simulink model "demo"  (R2016a)
settings: Solver=ode45  StartTime=0.0  StopTime=100  RelTol=1e-3
values from neighbouring files (symbols this model uses):
  P = computeGainsAerosonde(T_phi_delta_a,T_v_delta_r,T_theta_delta_e,T_Va_theta,T_Va_delta_t,P)    [run_autopilot.m]
  U_trim = [-0.0594; 0.0005; -0.0010; 0.0978]    [run_autopilot.m]
  x0 = X_trim    [run_autopilot.m]
  X_trim = [0; 0; -100.0000; 0.9993; -0.0011; 0.0332; 0.0186; 35.7388;             -0.0122; 2.3784; 0; 0; 0; -0.0300; 0; -0.0294; 0; 0.0978]    [run_autopilot.m]
undefined symbols (not defined in the file or in its folder): Earth, h_ref, lat0, lon0, T_elevon2ailelev, WGS84
undefined symbols (not defined in the file): param
libraries: simulink_extras x7, simulink x5, aerolibfltsims x4, X8_lib x3, aerolibactuator x3, aerolibanimutils x2, aerolibtransform2 x1, aerolibutil x1
settings Model: Creator=krisgry  LastModifiedBy=andreanv
settings DataIOCC: LimitDataPoints=on  SaveFormat=Array
settings DebuggingCC: AllowSymbolicDim=off
settings HardwareCC: ProdBitPerPointer=32  ProdLargestAtomicFloat=None  ProdIntDivRoundTo=Undefined  ProdEndianess=Unspecified  ProdWordSize=32  ProdHWDeviceType=32-bit Generic
settings ModelReferenceCC: PropagateSignalLabelsOutOfModel=off
settings ConfigComp: CovModelRefEnable=Off

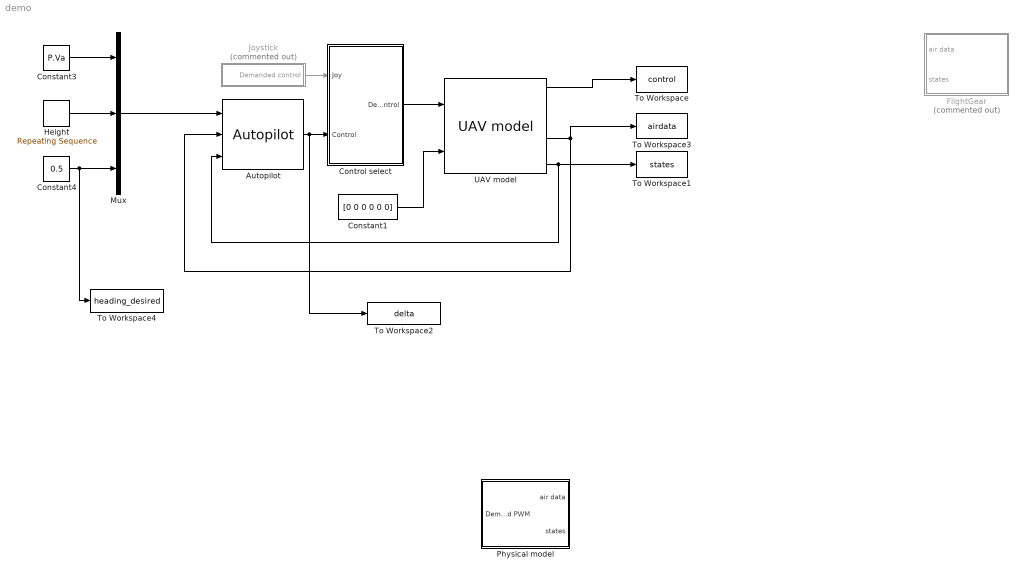
== system demo ==
  Autopilot : X8_lib/Autopilot  param=param  X_trim=X_trim  U_trim=U_trim
  Constant1 : Constant  Value=[0 0 0 0 0 0]
  Constant3 : Constant  Value=P.Va
  Constant4 : Constant  Value=0.5
  Control select : Subsystem
  FlightGear : Subsystem  Commented=on
  Height : simulink/Sources/Repeating Sequence  rep_seq_t=[0 1]  rep_seq_y=[-100 -100]
  Joystick : Subsystem  Commented=on
  Mux : Mux  Inputs=3
  Physical model : Subsystem
  To Workspace : ToWorkspace  VariableName=control  SaveFormat=Timeseries  SampleTime=-1
  To Workspace1 : ToWorkspace  VariableName=states  SaveFormat=Timeseries  SampleTime=-1
  To Workspace2 : ToWorkspace  VariableName=delta  SaveFormat=Timeseries  SampleTime=-1
  To Workspace3 : ToWorkspace  VariableName=airdata  SaveFormat=Timeseries  SampleTime=-1
  To Workspace4 : ToWorkspace  VariableName=heading_desired  SaveFormat=Timeseries  SampleTime=-1
  UAV model : X8_lib/UAV model  param=param  pos0=X_trim(1:3)'  quat0=X_trim(4:7)'  vel0=X_trim(8:10)'  rate0=X_trim(11:13)'  servoR_pos0=X_trim(14)  servoR_vel0=X_trim(15)  servoL_pos0=X_trim(16)  servoL_vel0=X_trim(17)  motor_speed0=X_trim(18)
  wires:
  Joystick/1(Demanded control) -> Control select/1(Joy)
  Autopilot/1 -> To Workspace2/1, Control select/2(Control)
  Mux/1 -> Autopilot/1
  Height/1 -> Mux/2
  Constant3/1 -> Mux/1
  Constant4/1 -> Mux/3, To Workspace4/1
  Control select/1(Demanded control) -> UAV model/1
  Constant1/1 -> UAV model/2
  UAV model/4 -> To Workspace1/1, Autopilot/3
  UAV model/3 -> To Workspace3/1, Autopilot/2
  UAV model/1 -> To Workspace/1

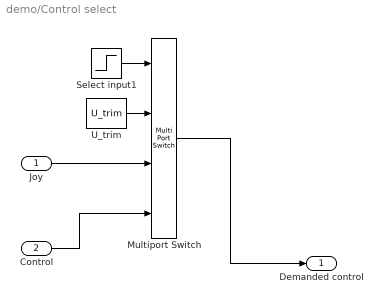
== system demo/Control select ==
  Joy : Inport
  Control : Inport  Port=2
  Multiport Switch : MultiPortSwitch
  Select input1 : Step  Time=0  Before=1  After=3  SampleTime=0
  U_trim : Constant  Value=U_trim
  Demanded control : Outport
  wires:
  Control/1 -> Multiport Switch/4
  Multiport Switch/1 -> Demanded control/1
  U_trim/1 -> Multiport Switch/2
  Joy/1 -> Multiport Switch/3
  Select input1/1 -> Multiport Switch/1

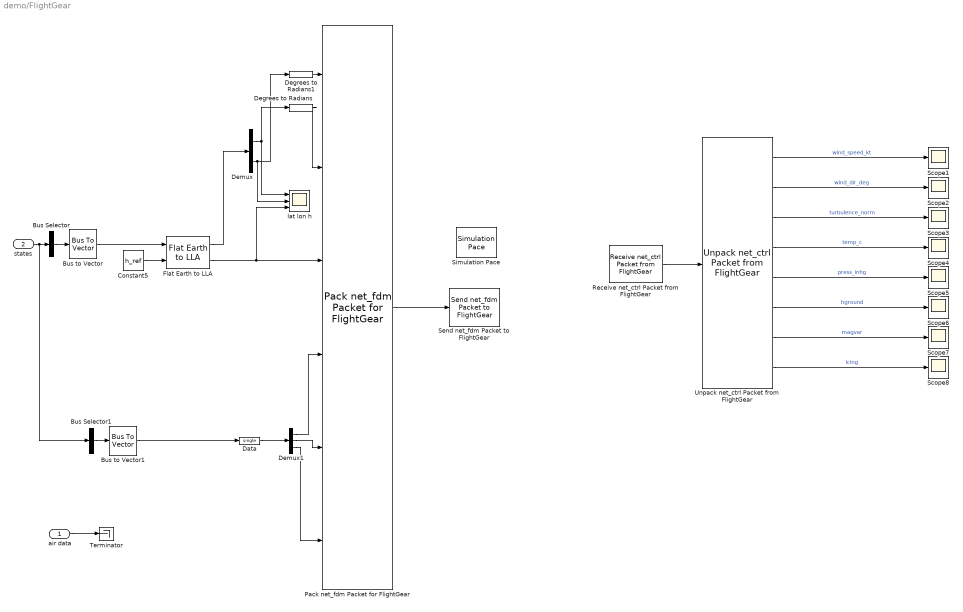
== system demo/FlightGear ==
  air data : Inport
  states : Inport  Port=2
  Bus Selector : BusSelector  OutputSignals=Position.p_N,Position.p_E,Position.p_D  OutputAsBus=on
  Bus Selector1 : BusSelector  OutputSignals=Attitude  OutputAsBus=on
  Bus to Vector : BusToVector
  Bus to Vector1 : BusToVector
  Constant5 : Constant  Value=h_ref
  Data : DataTypeConversion  OutDataTypeStr=single
  Degrees to Radians : simulink_extras/Transformations/Degrees to Radians
  Degrees to Radians1 : simulink_extras/Transformations/Degrees to Radians
  Demux : Demux  Outputs=2
  Demux1 : Demux  Outputs=3
  Flat Earth to LLA : aerolibtransform2/Flat Earth to LLA  units=Metric (MKS)  ptype=Earth (WGS84)  F=1/298.257223563  R=6378137  LL0=[lat0 lon0]  psi=0
  Pack net_fdm Packet for FlightGear : aerolibfltsims/Pack net_fdm Packet for FlightGear  FlightGearVersion=v2.12  ShowPositionAttitudeInputs=on  ShowVelocityAccelerationInputs=off  ShowControlSurfacePositionInputs=off  ShowEngineFuelInputs=off  ShowLandingGearInputs=off  ShowEnvironmentInputs=off  SampleTime=1/30
  Receive net_ctrl Packet from FlightGear : aerolibfltsims/Receive net_ctrl Packet from FlightGear  FlightGearVersion=v2.12  ReceiveAddress=129.241.154.119  ReceivePort=5505  ReceiveWidth=744  varLen=off  SampleTime=1/30  packetFlag=off
      settings: AttributesFormatString=Version Selected:\n%<FlightGearVersion>
  Scope{1..8} (8 alike) : Scope
  Send net_fdm Packet to FlightGear : aerolibfltsims/Send net_fdm Packet to FlightGear  DestinationIpAddress=129.241.154.119  DestinationPort=5502  LocalIpPort=-1  varLen=off  SampleTime=1/30
  Simulation Pace : aerolibanimutils/Simulation Pace  SimulationPace=1  SleepMode=MATLAB Thread  OutputPaceError=off  SampleTime=1/30
      settings: AttributesFormatString=%<SimulationPace> sec/sec
  Terminator : Terminator
  Unpack net_ctrl Packet from FlightGear : aerolibfltsims/Unpack net_ctrl Packet from FlightGear  FlightGearVersion=v2.12  ShowControlSurfacePositionOutputs=off  ShowEngineFuelOutputs=off  ShowLandingGearOutputs=off  ShowAvionicOutputs=off  ShowEnvironmentOutputs=on  SampleTime=1/30
      settings: AttributesFormatString=Version Selected: %<FlightGearVersion>
  lat lon h : Scope  NumInputPorts=3
  wires:
  Pack net_fdm Packet for FlightGear/1 -> Send net_fdm Packet to FlightGear/1
  Demux1/1 -> Pack net_fdm Packet for FlightGear/4
  Demux1/2 -> Pack net_fdm Packet for FlightGear/5
  Demux1/3 -> Pack net_fdm Packet for FlightGear/6
  Demux/2 -> lat lon h/2, Degrees to Radians1/1
  Demux/1 -> Degrees to Radians/1, lat lon h/1
  Data/1 -> Demux1/1
  Degrees to Radians/1 -> Pack net_fdm Packet for FlightGear/2
  Degrees to Radians1/1 -> Pack net_fdm Packet for FlightGear/1
  Unpack net_ctrl Packet from FlightGear/1 -> Scope1/1  "wind_speed_kt"
  Receive net_ctrl Packet from FlightGear/1 -> Unpack net_ctrl Packet from FlightGear/1
  Unpack net_ctrl Packet from FlightGear/2 -> Scope2/1  "wind_dir_deg"
  Unpack net_ctrl Packet from FlightGear/3 -> Scope3/1  "turbulence_norm"
  Unpack net_ctrl Packet from FlightGear/4 -> Scope4/1  "temp_c"
  Unpack net_ctrl Packet from FlightGear/5 -> Scope5/1  "press_inhg"
  Unpack net_ctrl Packet from FlightGear/6 -> Scope6/1  "hground"
  Unpack net_ctrl Packet from FlightGear/7 -> Scope7/1  "magvar"
  Unpack net_ctrl Packet from FlightGear/8 -> Scope8/1  "icing"
  air data/1 -> Terminator/1
  Constant5/1 -> Flat Earth to LLA/2
  Flat Earth to LLA/1 -> Demux/1
  Bus Selector/1 -> Bus to Vector/1
  Bus to Vector/1 -> Flat Earth to LLA/1
  Flat Earth to LLA/2 -> lat lon h/3, Pack net_fdm Packet for FlightGear/3
  Bus Selector1/1 -> Bus to Vector1/1
  Bus to Vector1/1 -> Data/1
  states/1 -> Bus Selector1/1, Bus Selector/1

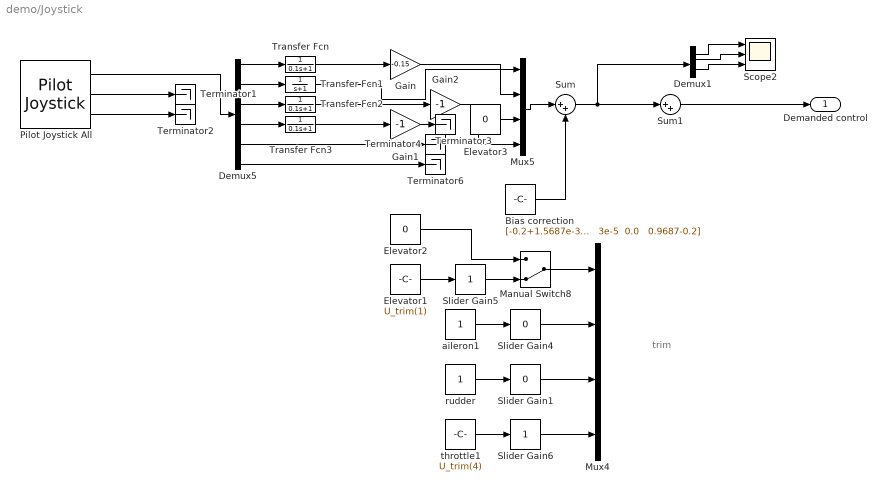
== system demo/Joystick ==
  note: trim
  Bias correction : Constant  Value="[-0.2+1.5687e-3   3e-5  0.0   0.9687-0.2]"
  Demux1 : Demux
  Demux5 : Demux  Outputs=6
  Elevator1 : Constant  Value=U_trim(1)
  Elevator2 : Constant  Value=0
  Elevator3 : Constant  Value=0
  Gain : Gain  Gain=-0.15
  Gain1 : Gain  Gain=-1
  Gain2 : Gain  Gain=-1
  Manual Switch8 : ManualSwitch  CurrentSetting=0
  Mux4 : Mux
  Mux5 : Mux
  Pilot Joystick All : aerolibanimutils/Pilot Joystick  JoystickID=Joystick1  OutputConfiguration=AllOutputs  SampleTime=1/30
  Scope2 : Scope  NumInputPorts=3
  Slider Gain1 : simulink/Math Operations/Slider Gain  low=-1  gain=0  high=1
  Slider Gain4 : simulink/Math Operations/Slider Gain  low=-1  gain=0  high=1
  Slider Gain5 : simulink/Math Operations/Slider Gain  low=-1  gain=1  high=1
  Slider Gain6 : simulink/Math Operations/Slider Gain  low=0  gain=1  high=2
  Sum : Sum  Inputs=|++
  Sum1 : Sum  Inputs=|++
  Terminator{1..4,6} (5 alike) : Terminator
  Transfer Fcn : TransferFcn  Denominator=[0.1 1]
  Transfer Fcn1 : TransferFcn  Denominator=[1 1]
  Transfer Fcn2 : TransferFcn  Denominator=[0.1 1]
  Transfer Fcn3 : TransferFcn  Denominator=[0.1 1]
  aileron1 : Constant
  rudder : Constant
  throttle1 : Constant  Value=U_trim(4)
  Demanded control : Outport
  wires:
  Gain/1 -> Mux5/2
  Demux5/5 -> Terminator4/1
  Demux5/1 -> Transfer Fcn/1
  Demux5/6 -> Terminator6/1
  Demux5/4 -> Transfer Fcn3/1
  Pilot Joystick All/3 -> Terminator2/1
  Pilot Joystick All/2 -> Terminator1/1
  Gain1/1 -> Terminator3/1
  Demux5/3 -> Transfer Fcn2/1
  Mux5/1 -> Sum/1
  Bias correction/1 -> Sum/2
  Gain2/1 -> Mux5/4
  Demux1/1 -> Scope2/1
  Demux1/2 -> Scope2/2
  Sum/1 -> Sum1/1, Demux1/1
  Elevator1/1 -> Slider Gain5/1
  aileron1/1 -> Slider Gain4/1
  Slider Gain4/1 -> Mux4/2
  Slider Gain6/1 -> Mux4/4
  Manual Switch8/1 -> Mux4/1
  Slider Gain5/1 -> Manual Switch8/2
  Elevator2/1 -> Manual Switch8/1
  Sum1/1 -> Demanded control/1
  throttle1/1 -> Slider Gain6/1
  Demux1/4 -> Scope2/3
  Elevator3/1 -> Mux5/3
  rudder/1 -> Slider Gain1/1
  Slider Gain1/1 -> Mux4/3
  Demux5/2 -> Transfer Fcn1/1
  Pilot Joystick All/1 -> Demux5/1
  Transfer Fcn/1 -> Gain/1
  Transfer Fcn1/1 -> Mux5/1
  Transfer Fcn2/1 -> Gain2/1
  Transfer Fcn3/1 -> Gain1/1

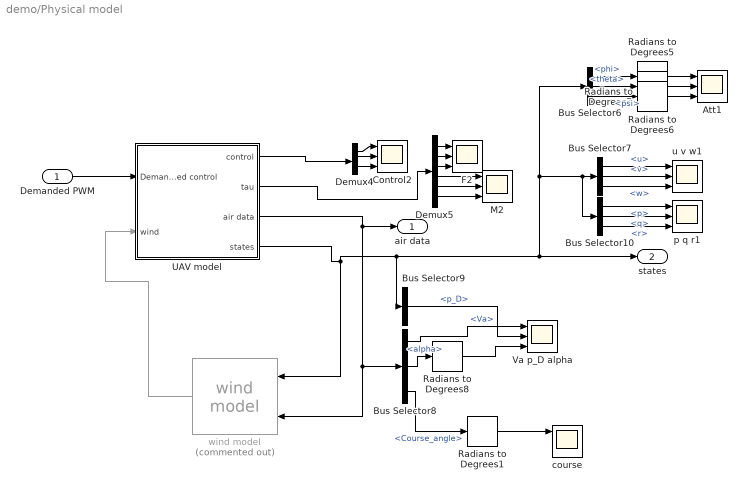
== system demo/Physical model ==
  Demanded PWM : Inport
  Att1 : Scope  NumInputPorts=3
  Bus Selector10 : BusSelector  OutputSignals=AngularVelocity.p,AngularVelocity.q,AngularVelocity.r
  Bus Selector6 : BusSelector  OutputSignals=Attitude.phi,Attitude.theta,Attitude.psi
  Bus Selector7 : BusSelector  OutputSignals=Velocity.u,Velocity.v,Velocity.w
  Bus Selector8 : BusSelector  OutputSignals=Va,alpha,Course_angle
  Bus Selector9 : BusSelector  OutputSignals=Position.p_D
  Control2 : Scope  NumInputPorts=3
  Demux4 : Demux
  Demux5 : Demux  Outputs=6
  F2 : Scope  NumInputPorts=3
  M2 : Scope  NumInputPorts=3
  Radians to Degrees{1,5..8} (5 alike) : simulink_extras/Transformations/Radians to Degrees
  UAV model : Subsystem  AncestorBlock=X8_lib/UAV model  mask{param=param, pos0=X_trim(1:3)', quat0=X_trim(4:7)', vel0=X_trim(8:10)', rate0=X_trim(11:13)', servoR_pos0=X_trim(14), servoR_vel0=X_trim(15), servoL_pos0=X_trim(16), servoL_vel0=X_trim(17), motor_speed0=X_trim(18)}
      mask prompts: param "UAV model"; pos0 "NED Position"; quat0 "Quaternion"; vel0 "Velocity"; rate0 "Angular Velocity"; servoR_pos0 "Right servo deflection"; servoR_vel0 "Right servo velocity"; servoL_pos0 "Left servo deflection"; servoL_vel0 "Left servo velocity"; motor_speed0 "Motor speed"
      mask help:
      | UAV model can be either 'x8_param' or 'aerosonde'
      |
      | # Inputs:
      | Demanded control: a 4x1 vector consisting of [elevator, aileron, rudder, throttle]
      | wind: a 6x1 vector consisting of the wind+gust in NED, and the body rate gusts: [N,E,D,p,q,r]
      |
      | # Outputs:
      | control: the control vector after it has been passed through the actuator model
      | tau: a 6x1 force/moment vector: [Fx,Fy,Fz,l,m,n]
      | airdata: a 10-element bus with airspeed, alpha, beta ... see bus_definitions.m
      | states: a bus consisting of 6 buses: position, attitude, quaternion, velocity, angular velocity, acceleration. See bus_definitions.m
      mask init:
      | %bus_defintions;
      | if(~exist('P') || ~isfield(P,'b'))
      |     init;
      | end
      mask DialogControl Container3 Prompt: Initial conditions
      mask Display:
      | image('X8.png')
      | port_label('output',1,'\delta','texmode','on')
      | port_label('output',2,'\tau','texmode','on')
      | port_label('output',3,'AirData','texmode','on')
      | port_label('output',4,'States','texmode','on')
      | port_label('input',1,'\delta_{demand}','texmode','on')
      | port_label('input',2,'Wind','texmode','on')
  Va p_D alpha : Scope  NumInputPorts=3
  course : Scope  NumInputPorts=3
  p q r1 : Scope  NumInputPorts=3
  u v w1 : Scope  NumInputPorts=3
  wind model : X8_lib/wind model  Commented=on  wind_speed=0  wind_dir=0  wind_start_time=0  param='x8_param'
  air data : Outport
  states : Outport  Port=2
  wires:
  Demux5/1 -> F2/1
  Demux5/2 -> F2/2
  Demux5/3 -> F2/3
  Demux5/4 -> M2/1
  Demux5/5 -> M2/2
  Demux5/6 -> M2/3
  Bus Selector7/1 -> u v w1/1  "<u>"
  Bus Selector7/2 -> u v w1/2  "<v>"
  Bus Selector7/3 -> u v w1/3  "<w>"
  Bus Selector6/1 -> Radians to Degrees5/1  "<phi>"
  Bus Selector6/3 -> Radians to Degrees7/1  "<psi>"
  Bus Selector6/2 -> Radians to Degrees6/1  "<theta>"
  Radians to Degrees5/1 -> Att1/1
  Radians to Degrees6/1 -> Att1/2
  Radians to Degrees7/1 -> Att1/3
  Bus Selector8/1 -> Va p_D alpha/1  "<Va>"
  Bus Selector9/1 -> Va p_D alpha/2  "<p_D>"
  Bus Selector8/2 -> Radians to Degrees8/1  "<alpha>"
  Radians to Degrees8/1 -> Va p_D alpha/3
  Demux4/4 -> Control2/3
  Demux4/2 -> Control2/2
  Demux4/1 -> Control2/1
  Bus Selector10/1 -> p q r1/1  "<p>"
  Bus Selector10/2 -> p q r1/2  "<q>"
  Bus Selector10/3 -> p q r1/3  "<r>"
  UAV model/3(air data) -> air data/1, wind model/2, Bus Selector8/1
  UAV model/4(states) -> wind model/1, Bus Selector9/1, Bus Selector6/1, Bus Selector7/1, Bus Selector10/1, states/1
  UAV model/2(tau) -> Demux5/1
  UAV model/1(control) -> Demux4/1
  wind model/1 -> UAV model/2(wind)
  Demanded PWM/1 -> UAV model/1(Demanded control)
  Bus Selector8/3 -> Radians to Degrees1/1  "<Course_angle>"
  Radians to Degrees1/1 -> course/1

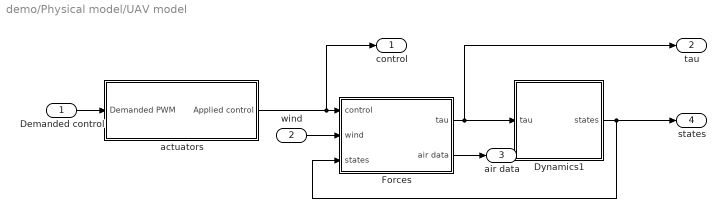
== system demo/Physical model/UAV model ==
  Demanded control : Inport
  wind : Inport  Port=2  PortDimensions=6
  Dynamics1 : Subsystem
  Forces : Subsystem
  actuators : Subsystem
  control : Outport
  tau : Outport  Port=2
  air data : Outport  Port=3  OutDataTypeStr=Bus: AirData
  states : Outport  Port=4  OutDataTypeStr=Bus: States
  wires:
  actuators/1(Applied control) -> Forces/1(control), control/1
  Forces/2(air data) -> air data/1
  Dynamics1/1(states) -> Forces/3(states), states/1
  Forces/1(tau) -> Dynamics1/1(tau), tau/1
  Demanded control/1 -> actuators/1(Demanded PWM)
  wind/1 -> Forces/2(wind)

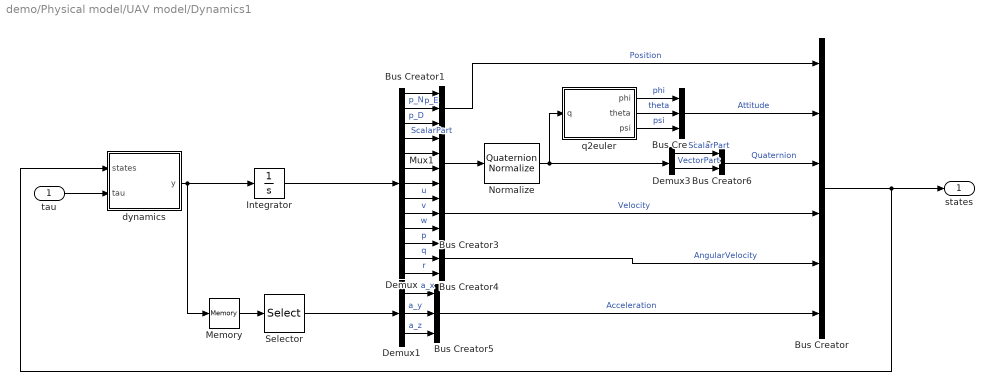
== system demo/Physical model/UAV model/Dynamics1 ==
  tau : Inport
  Bus Creator : BusCreator  Inputs=6  OutDataTypeStr=Bus: States
  Bus Creator1 : BusCreator  Inputs=3  OutDataTypeStr=Bus: Position
  Bus Creator2 : BusCreator  Inputs=3  OutDataTypeStr=Bus: Attitude
  Bus Creator3 : BusCreator  Inputs=3  OutDataTypeStr=Bus: Velocity
  Bus Creator4 : BusCreator  Inputs=3  OutDataTypeStr=Bus: AngularVelocity
  Bus Creator5 : BusCreator  Inputs=3  OutDataTypeStr=Bus: Acceleration
  Bus Creator6 : BusCreator  Inputs=2  OutDataTypeStr=Bus: Quaternion
  Demux : Demux  Outputs=13
  Demux1 : Demux  Outputs=3
  Demux3 : Demux  Outputs=[1,3]
  Integrator : Integrator  InitialCondition=[pos0,quat0,vel0,rate0]%x0(1:13)
  Memory : Memory
  Mux1 : Mux
  Normalize : aerolibutil/Quaternion Normalize
  Selector : Selector  InputPortWidth=13  IndexOptions=Index vector (dialog)  Indices=8:10  OutputSizes=1
  dynamics : MATLAB Function  TreatAsAtomicUnit=on
  q2euler : MATLAB Function  TreatAsAtomicUnit=on
  states : Outport
  wires:
  Memory/1 -> Selector/1
  Mux1/1 -> Normalize/1
  Bus Creator2/1 -> Bus Creator/2  "Attitude"
  Demux/4 -> Mux1/1  "ScalarPart"
  Bus Creator6/1 -> Bus Creator/3  "Quaternion"
  Demux3/2 -> Bus Creator6/2  "VectorPart"
  Demux3/1 -> Bus Creator6/1  "ScalarPart"
  Integrator/1 -> Demux/1
  Normalize/1 -> Demux3/1, q2euler/1(q)
  Demux/5 -> Mux1/2
  Demux/7 -> Mux1/4
  Demux/6 -> Mux1/3
  Demux1/3 -> Bus Creator5/3  "a_z"
  Demux1/2 -> Bus Creator5/2  "a_y"
  Demux1/1 -> Bus Creator5/1  "a_x"
  Selector/1 -> Demux1/1
  Bus Creator5/1 -> Bus Creator/6  "Acceleration"
  Bus Creator4/1 -> Bus Creator/5  "AngularVelocity"
  Bus Creator1/1 -> Bus Creator/1  "Position"
  Bus Creator3/1 -> Bus Creator/4  "Velocity"
  Demux/12 -> Bus Creator4/2  "q"
  Demux/13 -> Bus Creator4/3  "r"
  Demux/11 -> Bus Creator4/1  "p"
  Demux/9 -> Bus Creator3/2  "v"
  Demux/8 -> Bus Creator3/1  "u"
  Demux/10 -> Bus Creator3/3  "w"
  q2euler/1(phi) -> Bus Creator2/1  "phi"
  q2euler/3(psi) -> Bus Creator2/3  "psi"
  q2euler/2(theta) -> Bus Creator2/2  "theta"
  Demux/1 -> Bus Creator1/1  "p_N"
  Demux/3 -> Bus Creator1/3  "p_D"
  Demux/2 -> Bus Creator1/2  "p_E"
  Bus Creator/1 -> dynamics/1(states), states/1
  tau/1 -> dynamics/2(tau)
  dynamics/1(y) -> Integrator/1, Memory/1

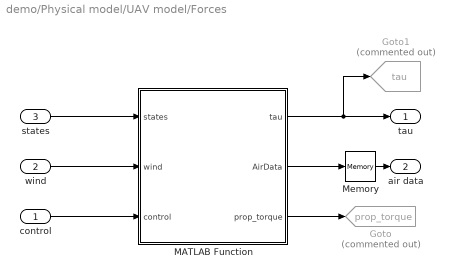
== system demo/Physical model/UAV model/Forces ==
  control : Inport
  wind : Inport  Port=2
  states : Inport  Port=3
  Goto : Goto  Commented=on  GotoTag=prop_torque  TagVisibility=global
  Goto1 : Goto  Commented=on  GotoTag=tau  TagVisibility=global
  MATLAB Function : MATLAB Function  TreatAsAtomicUnit=on
  Memory : Memory  X0=1e-15
  tau : Outport
  air data : Outport  Port=2
  wires:
  MATLAB Function/2(AirData) -> Memory/1
  Memory/1 -> air data/1
  MATLAB Function/3(prop_torque) -> Goto/1
  MATLAB Function/1(tau) -> tau/1, Goto1/1
  wind/1 -> MATLAB Function/2(wind)
  control/1 -> MATLAB Function/3(control)
  states/1 -> MATLAB Function/1(states)

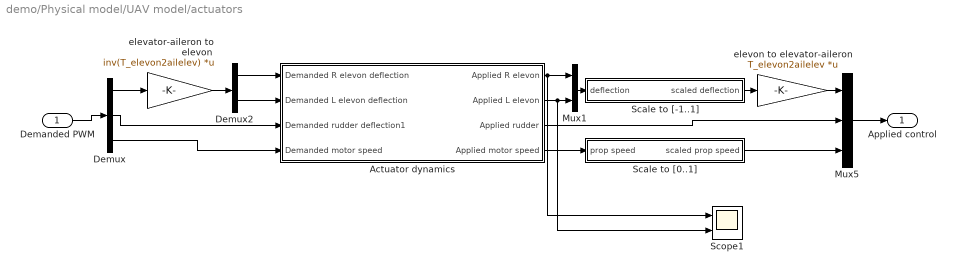
== system demo/Physical model/UAV model/actuators ==
  Demanded PWM : Inport
  Actuator dynamics : Subsystem
  Demux : Demux  Outputs=[2,1,1]
  Demux2 : Demux  Outputs=2
  Mux1 : Mux  Inputs=2
  Mux5 : Mux  Inputs=3
  Scale to [-1..1] : Subsystem
  Scale to [0..1] : Subsystem
  Scope1 : Scope  NumInputPorts=2
  elevator-aileron to elevon : Gain  Gain=inv(T_elevon2ailelev)  Multiplication=Matrix(K*u) (u vector)
  elevon to elevator-aileron : Gain  Gain=T_elevon2ailelev  Multiplication=Matrix(K*u) (u vector)
  Applied control : Outport
  wires:
  Demux/3 -> Actuator dynamics/4(Demanded motor speed)
  Mux5/1 -> Applied control/1
  Demux/2 -> Actuator dynamics/3(Demanded rudder deflection1)
  Mux1/1 -> Scale to [-1..1]/1(deflection)
  Actuator dynamics/1(Applied R elevon) -> Mux1/1, Scope1/1
  Scale to [0..1]/1(scaled prop speed) -> Mux5/3
  Actuator dynamics/3(Applied rudder) -> Mux5/2
  elevon to elevator-aileron/1 -> Mux5/1
  Scale to [-1..1]/1(scaled deflection) -> elevon to elevator-aileron/1
  Actuator dynamics/4(Applied motor speed) -> Scale to [0..1]/1(prop speed)
  Actuator dynamics/2(Applied L elevon) -> Mux1/2, Scope1/2
  Demux2/1 -> Actuator dynamics/1(Demanded R elevon deflection)
  Demux/1 -> elevator-aileron to elevon/1
  elevator-aileron to elevon/1 -> Demux2/1
  Demux2/2 -> Actuator dynamics/2("Demanded L elevon deflection ")
  Demanded PWM/1 -> Demux/1

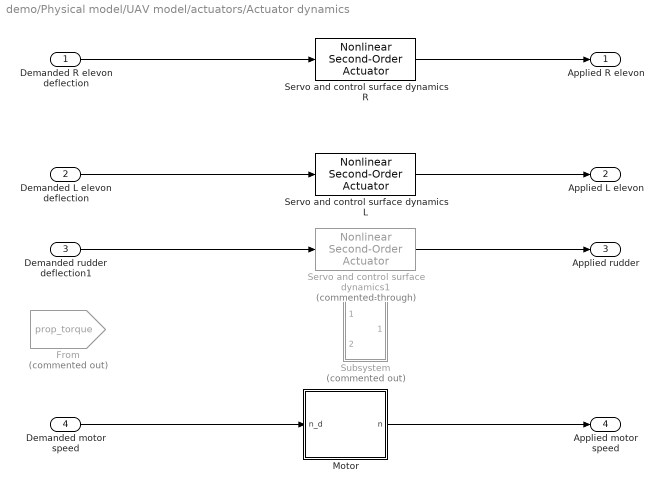
== system demo/Physical model/UAV model/actuators/Actuator dynamics ==
  Demanded R elevon deflection : Inport
  "Demanded L elevon deflection " : Inport  Port=2
  Demanded rudder deflection1 : Inport  Port=3
  Demanded motor speed : Inport  Port=4
  From : From  Commented=on  GotoTag=prop_torque  TagVisibility=global
  Motor : Subsystem  mask{T=0.2, X0=motor_speed0}
      mask prompts: T "Time constant"; X0 "Initial condition"
      mask DialogControl DescTextVar Prompt: Simple first order motor model
  Servo and control surface dynamics L : aerolibactuator/Nonlinear Second-Order Actuator  wn_fin=P.servo.omega0  z_fin=P.servo.zeta  fin_max=P.servo.max_rad  fin_min=P.servo.min_rad  fin_maxrate=P.servo.rate_lim  fin_act_0=servoL_pos0  fin_act_vel=servoL_vel0
  Servo and control surface dynamics R : aerolibactuator/Nonlinear Second-Order Actuator  wn_fin=P.servo.omega0  z_fin=P.servo.zeta  fin_max=P.servo.max_rad  fin_min=P.servo.min_rad  fin_maxrate=P.servo.rate_lim  fin_act_0=servoR_pos0  fin_act_vel=servoR_vel0
  Servo and control surface dynamics1 : aerolibactuator/Nonlinear Second-Order Actuator  Commented=through  wn_fin=P.servo.omega0  z_fin=P.servo.zeta  fin_max=P.servo.max_rad  fin_min=P.servo.min_rad  fin_maxrate=P.servo.rate_lim  fin_act_0=P.servo.pos0  fin_act_vel=P.servo.rate0
  Subsystem : Subsystem  Commented=on
  Applied R elevon : Outport
  Applied L elevon : Outport  Port=2
  Applied rudder : Outport  Port=3
  Applied motor speed : Outport  Port=4
  wires:
  Demanded motor speed/1 -> Motor/1(n_d)
  Demanded rudder deflection1/1 -> Servo and control surface dynamics1/1
  "Demanded L elevon deflection "/1 -> Servo and control surface dynamics L/1
  Demanded R elevon deflection/1 -> Servo and control surface dynamics R/1
  Servo and control surface dynamics L/1 -> Applied L elevon/1
  Servo and control surface dynamics1/1 -> Applied rudder/1
  Motor/1(n) -> Applied motor speed/1
  Servo and control surface dynamics R/1 -> Applied R elevon/1

== system demo/Physical model/UAV model/actuators/Scale to [-1..1] ==
  deflection : Inport
  Gain : Gain  Gain=P.rad2unit
  Saturation : Saturate  UpperLimit=1  LowerLimit=-1
  scaled deflection : Outport
  wires:
  Saturation/1 -> scaled deflection/1
  Gain/1 -> Saturation/1
  deflection/1 -> Gain/1

== system demo/Physical model/UAV model/actuators/Scale to [0..1] ==
  prop speed : Inport
  Gain : Gain  Commented=through  Gain=1/P.motor.omega_max
  Saturation : Saturate  UpperLimit=1  LowerLimit=0
  scaled prop speed : Outport
  wires:
  Saturation/1 -> scaled prop speed/1
  Gain/1 -> Saturation/1
  prop speed/1 -> Gain/1

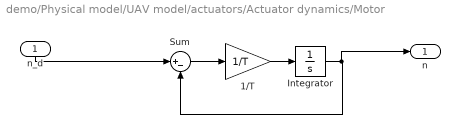
== system demo/Physical model/UAV model/actuators/Actuator dynamics/Motor ==
  n_d : Inport
  1/T : Gain  Gain=1/T
  Integrator : Integrator  InitialCondition=X0  ContinuousStateAttributes='throttle'
  Sum : Sum  Inputs=|+-
  n : Outport
  wires:
  1/T/1 -> Integrator/1
  Sum/1 -> 1/T/1
  n_d/1 -> Sum/1
  Integrator/1 -> Sum/2, n/1

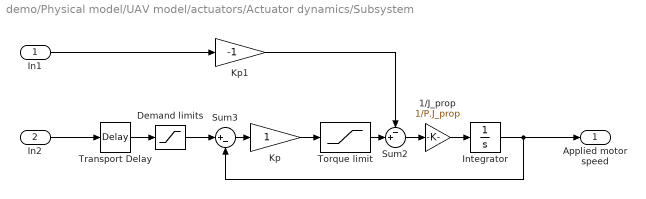
== system demo/Physical model/UAV model/actuators/Actuator dynamics/Subsystem ==
  In1 : Inport
  In2 : Inport  Port=2
  1/J_prop : Gain  Gain=1/P.J_prop  SaturateOnIntegerOverflow=on  OutDataTypeStr=Inherit: Same as input  ParamDataTypeStr=Inherit: Same as input
  Demand limits : Saturate  UpperLimit=1  LowerLimit=0
  Integrator : Integrator  InitialCondition=0.5
  Kp : Gain  SaturateOnIntegerOverflow=on  OutDataTypeStr=Inherit: Same as input  ParamDataTypeStr=Inherit: Same as input
  Kp1 : Gain  Gain=-1  SaturateOnIntegerOverflow=on  OutDataTypeStr=Inherit: Same as input  ParamDataTypeStr=Inherit: Same as input
  Sum2 : Sum  Inputs=-+|  SaturateOnIntegerOverflow=on  InputSameDT=on  OutDataTypeStr=Inherit: Same as first input
  Sum3 : Sum  Inputs=|+-  SaturateOnIntegerOverflow=on  InputSameDT=on  OutDataTypeStr=Inherit: Same as first input
  Torque limit : Saturate  UpperLimit=P.motor.torque_max  LowerLimit=0  ZeroCross=off
  Transport Delay : TransportDelay  DelayTime=0.001  PadeOrder=1
  Applied motor speed : Outport
  wires:
  Kp1/1 -> Sum2/1
  Transport Delay/1 -> Demand limits/1
  In2/1 -> Transport Delay/1
  In1/1 -> Kp1/1
  Kp/1 -> Torque limit/1
  1/J_prop/1 -> Integrator/1
  Sum2/1 -> 1/J_prop/1
  Torque limit/1 -> Sum2/2
  Integrator/1 -> Sum3/2, Applied motor speed/1
  Sum3/1 -> Kp/1
  Demand limits/1 -> Sum3/1

== matlab function demo/Physical model/UAV model/Forces/MATLAB Function ==
  data: states input; tau output; AirData output Bus: AirData; wind input; control input; P parameter; prop_torque output
function [tau,AirData,prop_torque]  = fcn(states,wind,control,P)
%#codegen
% ,Va, alpha, beta, course, crab, gamma, gamma_a, wind_b,T_prop
temp = forces([states.Position.p_N,states.Position.p_E,states.Position.p_D,states.Attitude.phi,states.Attitude.theta,states.Attitude.psi]',...
              [states.Velocity.u,states.Velocity.v,states.Velocity.w,states.AngularVelocity.p,states.AngularVelocity.q,states.AngularVelocity.r]',...
              [states.Quaternion.ScalarPart;states.Quaternion.VectorPart]',control,wind,P);
tau = temp(1:6);
AirData.Va                              = temp(7);
AirData.alpha                           = temp(8);
AirData.beta                            = temp(9);
AirData.Course_angle                    = temp(10);
AirData.Crab_angle                      = temp(11);
AirData.Path_angle                      = temp(12);
AirData.Air_mass_referenced_path_angle  = temp(13);
AirData.wind_x                          = temp(14);
AirData.wind_y                          = temp(15);
AirData.wind_z                          = temp(16);

prop_torque     = temp(17);

== matlab function demo/Physical model/UAV model/Dynamics1/q2euler ==
  data: q input; phi output; theta output; psi output
function [phi,theta,psi] = fcn(q)
%#codegen
[phi,theta,psi] = q2euler(q);
end

== matlab function demo/Physical model/UAV model/Dynamics1/dynamics ==
  data: states input Bus: States; tau input; y output; P parameter
function y = fcn(states,tau, P)
%#codegen

y = dynamics([states.Position.p_N,states.Position.p_E,states.Position.p_D]',[states.Quaternion.ScalarPart,states.Quaternion.VectorPart']',...
       [states.Velocity.u,states.Velocity.v,states.Velocity.w]',[states.AngularVelocity.p,states.AngularVelocity.q,states.AngularVelocity.r]',...
       tau,P);
% y = dynamics(states(1:3),states(4:7),states(8:10),states(11:13),tau,P);
end
